simulink model "IsourceTest"  (Simulink 8.1)
settings: Solver=FixedStepDiscrete  StartTime=0.0  StopTime=2  FixedStep=Ts  RelTol=1e-3
undefined symbols (not defined in the file or in its folder): D1, Delta, DiscIntNeverNeededParam, sigbuilder_block, Ts
libraries: powerlib x8, breaker_lib x2, IsourcePower_lib x1
settings Model: Creator=pkoralew  LastModifiedBy=pkoralew
settings DebuggingCC: FcnCallInpInsideContextMsg=EnableAllAsWarning

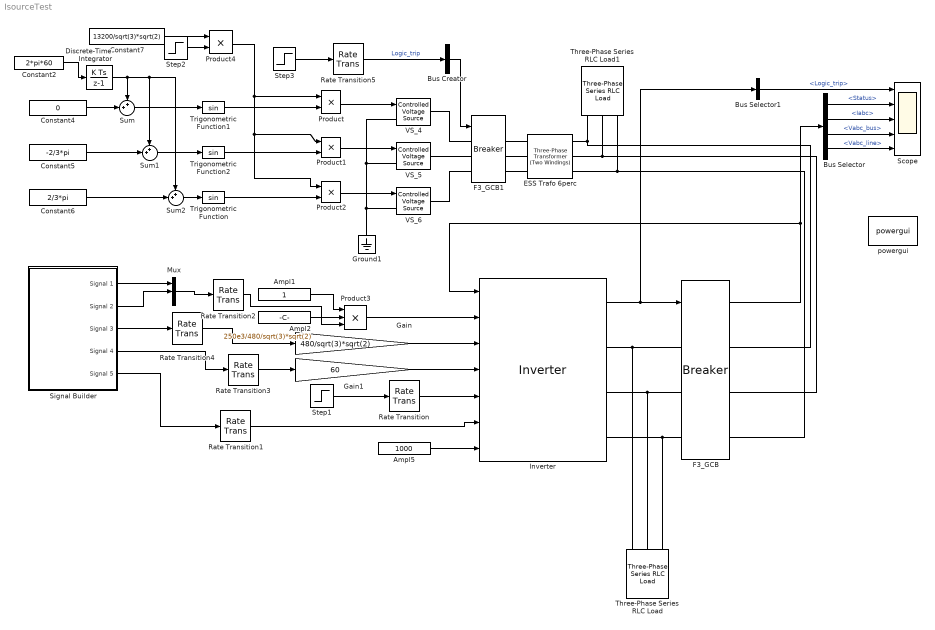
== system IsourceTest ==
  Ampl1 : Constant
  Ampl2 : Constant  Value=250e3/480/sqrt(3)*sqrt(2)
  Ampl5 : Constant  Value=1000
  Bus Creator : BusCreator  Inputs=1
  Bus Selector : BusSelector  OutputSignals=Status,Iabc,Vabc_bus,Vabc_line
  Bus Selector1 : BusSelector  OutputSignals=Logic_trip
  Constant2 : Constant  Value=2*pi*60
  Constant4 : Constant  Value=0
  Constant5 : Constant  Value=-2/3*pi
  Constant6 : Constant  Value=2/3*pi
  Constant7 : Constant  Value=13200/sqrt(3)*sqrt(2)
  Discrete-Time Integrator : DiscreteIntegrator  SampleTime=Ts  ICPrevOutput=DiscIntNeverNeededParam  ICPrevScaledInput=DiscIntNeverNeededParam
  ESS Trafo 6perc : powerlib/Elements/Three-Phase Transformer (Two Windings)  Winding1Connection=Yg  UNITS=pu  NominalPower=[250e3 60]  Winding1=[480 0.003 0.03]  Winding2Connection=Delta (D1)  Winding2=[13200 0.003 0.03]  SetSaturation=off  Rm=100  Lm=100  Saturation=[0 0;0.0031999 1.2;1.3333 1.52]  Hysteresis=off  DataFile='hysteresis'  SetInitialFlux=off  InitialFluxes=[0.79999 -0.79999 0.70002]  Measurements=Fluxes and magnetization currents ( Imag )  MoreParameters=off  BreakLoop=off  DataType=off  TransfoNumber=1
  F3_GCB : breaker_lib/Breaker  Ts=Ts  mech_delay=cb_mech_delay
  F3_GCB1 : breaker_lib/Breaker  Ts=Ts  mech_delay=cb_mech_delay
  Gain : Gain  Gain=480/sqrt(3)*sqrt(2)
  Gain1 : Gain  Gain=60
  Ground1 : powerlib/Elements/Ground  LConnTagsString=a
  Inverter : IsourcePower_lib/Inverter
  Mux : Mux  Inputs=3
  Product : Product  RndMeth=Zero
  Product1 : Product  RndMeth=Zero
  Product2 : Product  RndMeth=Zero
  Product3 : Product  Inputs=3  RndMeth=Zero
  Product4 : Product
  Rate Transition{,1..5} (6 alike) : RateTransition
  Scope : Scope  NumInputPorts=5
      settings: YMin=-5~-5~-5~-5~-5  YMax=5~5~5~5~5
  Signal Builder : Subsystem  Tag=STV Subsys  LoadFcn=sigbuilder_block('load');  StartFcn=sigbuilder_block('start');  StopFcn=sigbuilder_block('stop');  ClipboardFcn=sigbuilder_block('clipboard');  mask(Sigbuilder block){}
      mask help: Sigbuilder GUI
      mask init:
      | if ~strcmp(get_param(bdroot(gcbh),'SimulationStatus'),'stopped') tuvar = sigbuilder_block('maskInit'); end
      settings: CopyFcn=sigbuilder_block('copy');  DeleteFcn=sigbuilder_block('delete');  ModelCloseFcn=sigbuilder_block('modelClose');  PreSaveFcn=sigbuilder_block('preSave');  PauseFcn=sigbuilder_block('pause')  ContinueFcn=sigbuilder_block('continue')  NameChangeFcn=sigbuilder_block('namechange');  OpenFcn=sigbuilder_block('open',[5.58621 9.31034 1031.59 587.793 ]);  CloseFcn=sigbuilder_block('close');
      mask Display: plot(0,0,100,100,[10,10,40,40,10],[80,20,20,80,80],[40,10],[50,50], [40,27,10],[65,72,56],[40,25,25,10],[28,28,43,43]);
  Step1 : Step  SampleTime=0
  Step2 : Step  Time=0.001  SampleTime=0
  Step3 : Step  Before=1  After=0  SampleTime=0
  Sum : Sum  Inputs=++|
  Sum1 : Sum  Inputs=++|
  Sum2 : Sum  Inputs=++|
  Three-Phase Series RLC Load : powerlib/Elements/Three-Phase Series RLC Load  LConnTagsString=A|B|C  Configuration=Delta  NominalVoltage=480  NominalFrequency=60  ActivePower=1e3  InductivePower=0  CapacitivePower=100  Measurements=None  LoadType=constant Z
  Three-Phase Series RLC Load1 : powerlib/Elements/Three-Phase Series RLC Load  LConnTagsString=A|B|C  Configuration=Delta  NominalVoltage=480  NominalFrequency=60  ActivePower=1e3  InductivePower=0  CapacitivePower=100  Measurements=None  LoadType=constant Z
  Trigonometric Function : Trigonometry
  Trigonometric Function1 : Trigonometry
  Trigonometric Function2 : Trigonometry
  VS_4 : powerlib/Electrical Sources/Controlled Voltage Source  Initialize=off  Source_Type=AC  Amplitude=0  Phase=0  Frequency=0  Measurements=None
  VS_5 : powerlib/Electrical Sources/Controlled Voltage Source  Initialize=off  Source_Type=AC  Amplitude=0  Phase=0  Frequency=0  Measurements=None
  VS_6 : powerlib/Electrical Sources/Controlled Voltage Source  Initialize=off  Source_Type=AC  Amplitude=0  Phase=0  Frequency=0  Measurements=None
  powergui : powerlib/powergui  Priority=1  SimulationMode=Discrete  SolverType=Tustin  SampleTime=Ts  frequency=60  SPID=off  DisableSnubberDevices=off  DisableRonSwitches=off  DisableVfSwitches=off  SwTol=0  Interpol=off  DisplayEquations=off  frequencyindice=0  Pbase=100e6  ErrMax=1e-4  Iterations=50  UnitsV=kV  UnitsW=MW  FunctionMessages=off  echomessages=off  HookPort=off  EnableUseOfTLC=off  x0status=blocks  RestoreLinks=warning  ResistiveCurrentMeasurement=off  Frange=[0:2:500]  Ylog=off  Xlog=on  ShowGrid=off  save=off  variable=ZData  ZoomFFT=off  StartTime=0.0  cycles=1  DisplayStyle=1  fundamental=60  FreqAxis=off  MaxFrequency=1000  frequencyindicesteady=1  RmsSteady=1  display=off  Ts=0  methode=off
  wires:
  Product4/1 -> Product1/1, Product2/1, Product/1
  Trigonometric Function1/1 -> Product/2
  Discrete-Time Integrator/1 -> Sum2/1, Sum1/1, Sum/1
  Sum/1 -> Trigonometric Function1/1
  Sum1/1 -> Trigonometric Function2/1
  Constant2/1 -> Discrete-Time Integrator/1
  Constant4/1 -> Sum/2
  Sum2/1 -> Trigonometric Function/1
  Constant5/1 -> Sum1/2
  Constant6/1 -> Sum2/2
  Trigonometric Function2/1 -> Product1/2
  Trigonometric Function/1 -> Product2/2
  Product/1 -> VS_4/1
  Product1/1 -> VS_5/1
  Product2/1 -> VS_6/1
  Ampl2/1 -> Product3/2
  Ampl1/1 -> Product3/1
  Product3/1 -> Inverter/2
  Signal Builder/5(Signal 5) -> Rate Transition1/1
  Step1/1 -> Rate Transition/1
  Gain1/1 -> Inverter/4
  Constant7/1 -> Product4/1
  Step2/1 -> Product4/2
  Inverter/1 -> Bus Selector1/1, F3_GCB/1
  F3_GCB/1 -> Bus Selector/1, Inverter/1
  Bus Selector1/1 -> Scope/1  "<Logic_trip>"
  Bus Selector/2 -> Scope/3  "<Iabc>"
  Bus Selector/1 -> Scope/2  "<Status>"
  Bus Selector/4 -> Scope/5  "<Vabc_line>"
  Bus Selector/3 -> Scope/4  "<Vabc_bus>"
  Rate Transition/1 -> Inverter/5
  Rate Transition1/1 -> Inverter/6
  Rate Transition2/1 -> Product3/3
  Ampl5/1 -> Inverter/7
  Gain/1 -> Inverter/3
  Mux/1 -> Rate Transition2/1
  Signal Builder/1(Signal 1) -> Mux/1
  Signal Builder/2(Signal 2) -> Mux/2
  Signal Builder/3(Signal 3) -> Rate Transition4/1
  Signal Builder/4(Signal 4) -> Rate Transition3/1
  Rate Transition3/1 -> Gain1/1
  Rate Transition4/1 -> Gain/1
  Rate Transition5/1 -> Bus Creator/1  "Logic_trip"
  Step3/1 -> Rate Transition5/1
  Bus Creator/1 -> F3_GCB1/1
  connections:
  Ground1/LConn1 -- VS_6/LConn1 -- VS_5/LConn1 -- VS_4/LConn1
  ESS Trafo 6perc/LConn2 -- F3_GCB/RConn2 -- Three-Phase Series RLC Load1/LConn2
  ESS Trafo 6perc/LConn3 -- F3_GCB/RConn3 -- Three-Phase Series RLC Load1/LConn3
  ESS Trafo 6perc/LConn1 -- F3_GCB/RConn1 -- Three-Phase Series RLC Load1/LConn1
  Three-Phase Series RLC Load/LConn1 -- Inverter/RConn1 -- F3_GCB/LConn1
  Three-Phase Series RLC Load/LConn2 -- Inverter/RConn2 -- F3_GCB/LConn2
  Three-Phase Series RLC Load/LConn3 -- Inverter/RConn3 -- F3_GCB/LConn3
  VS_4/RConn1 -- F3_GCB1/LConn1
  F3_GCB1/LConn2 -- VS_5/RConn1
  F3_GCB1/LConn3 -- VS_6/RConn1
  F3_GCB1/RConn1 -- ESS Trafo 6perc/RConn1
  F3_GCB1/RConn2 -- ESS Trafo 6perc/RConn2
  F3_GCB1/RConn3 -- ESS Trafo 6perc/RConn3

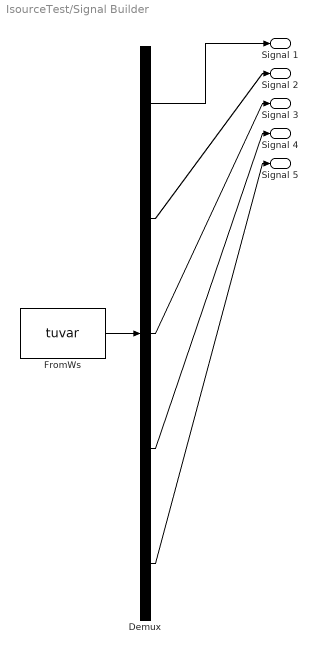
== system IsourceTest/Signal Builder ==
  Demux : Demux  Tag=STV Demux  Outputs=5
  FromWs : FromWorkspace  Tag=STV FromWs  VariableName=tuvar  SampleTime=0  SigBuilderData=DataTag0  VnvData=DataTag1
      SigBuilderData=|
      | common.afterFinalStr = 'Extrapolate'
      | common.sampleTime = 0
      | dataSet(1).timeRange = [0 2]
      | dataSet(1).name = 'Group 2'
      | dataSet(2).timeRange = [0 0.4]
      | dataSet(2).name = 'Group 3'
      | dataSet(3).timeRange = [0 0.4]
      | dataSet(3).name = 'Group 4'
      | dataSet(4).timeRange = [0 0.4]
      | dataSet(4).name = 'Group 5'
      | dataSet(5).timeRange = [0 0.4]
      | dataSet(5).name = 'Group 6'
      | sbobj.Groups(1).Name = 'Group 2'
      | sbobj.Groups(1).Signals(1).Name = 'Signal 1'
      | sbobj.Groups(1).Signals(1).XData = [0 0.3 0.385 0.455 0.532 0.634 0.634 0.746 0.746 0.85 2]
      | sbobj.Groups(1).Signals(1).YData = [0 0 1 1 0 0 -1 -1 0 0 0]
      | sbobj.Groups(1).Signals(2).Name = 'Signal 2'
      | sbobj.Groups(1).Signals(2).XData = [0 0.33 0.5 0.59 0.7 0.806 2]
      | sbobj.Groups(1).Signals(2).YData = [0 0 1 1 -1 0 0]
      | sbobj.Groups(1).Signals(3).Name = 'Signal 3'
      | sbobj.Groups(1).Signals(3).XData = [0 1 1 1.202 1.202 2]
      | sbobj.Groups(1).Signals(3).YData = [1 1 0.71 0.71 1.39 1.39]
      | sbobj.Groups(1).Signals(4).Name = 'Signal 4'
      | sbobj.Groups(1).Signals(4).XData = [0 1.202 1.202 1.396 1.396 2]
      | sbobj.Groups(1).Signals(4).YData = [1 1 0.95 0.95 1.048 1.048]
      | sbobj.Groups(1).Signals(5).Name = 'Signal 5'
      | sbobj.Groups(1).Signals(5).XData = [0 0.042 0.042 1.488 1.488 1.636 1.636 2]
      | sbobj.Groups(1).Signals(5).YData = [0 0 1 1 0 0 1 1]
      | sbobj.Groups(1).TimeRange = [0 2]
      | sbobj.Groups(2).Name = 'Group 3'
      | sbobj.Groups(2).Signals(1).Name = 'Signal 1'
      | sbobj.Groups(2).Signals(1).XData = [0 0.005 0.03 0.041 0.0445 0.0575 0.0675 0.0785 0.0905 0.0945 0.1055 0.1115 0.133 0.1455 0.1565 0.1635 0.192 0.218 0.306 0.3075 0.4]
      | sbobj.Groups(2).Signals(1).YData = [0 0 0.5 0.5 0.382 0.384 0.7 0.702 0.918 0.482 0.482 1 1 0.606 0.74 0.35 0.672 0.014 0.398 0.202 0]
      | sbobj.Groups(2).Signals(2).Name = 'Signal 2'
      | sbobj.Groups(2).Signals(2).XData = [0 0.16 0.16 0.24 0.24 10]
      | sbobj.Groups(2).Signals(2).YData = [0 0 1 1 0 0]
      | sbobj.Groups(2).Signals(3).Name = 'Signal 3'
      | sbobj.Groups(2).Signals(3).XData = [0 1 1 10]
      | sbobj.Groups(2).Signals(3).YData = [0 0 1 1]
      | sbobj.Groups(2).Signals(4).Name = 'Signal 4'
      | sbobj.Groups(2).Signals(4).XData = [0 1 1 10]
      | sbobj.Groups(2).Signals(4).YData = [0 0 1 1]
      | sbobj.Groups(2).Signals(5).Name = 'Signal 5'
      | sbobj.Groups(2).Signals(5).XData = [0 1 1 10]
      | sbobj.Groups(2).Signals(5).YData = [0 0 1 1]
      | sbobj.Groups(3).Name = 'Group 4'
      | sbobj.Groups(3).Signals(1).Name = 'Signal 1'
      | sbobj.Groups(3).Signals(1).XData = [0 0.1 0.1 0.2 0.2 0.4]
      | sbobj.Groups(3).Signals(1).YData = [0 0 0.5 0.5 0 0]
      | sbobj.Groups(3).Signals(2).Name = 'Signal 2'
      | sbobj.Groups(3).Signals(2).XData = [0 0.16 0.16 0.24 0.24 10]
      | sbobj.Groups(3).Signals(2).YData = [0 0 1 1 0 0]
      | sbobj.Groups(3).Signals(3).Name = 'Signal 3'
      | sbobj.Groups(3).Signals(3).XData = [0 1 1 10]
      | sbobj.Groups(3).Signals(3).YData = [0 0 1 1]
      | sbobj.Groups(3).Signals(4).Name = 'Signal 4'
      | sbobj.Groups(3).Signals(4).XData = [0 1 1 10]
      | sbobj.Groups(3).Signals(4).YData = [0 0 1 1]
      | sbobj.Groups(3).Signals(5).Name = 'Signal 5'
      | sbobj.Groups(3).Signals(5).XData = [0 1 1 10]
      | sbobj.Groups(3).Signals(5).YData = [0 0 1 1]
      | sbobj.Groups(4).Name = 'Group 5'
      | sbobj.Groups(4).Signals(1).Name = 'Signal 1'
      | sbobj.Groups(4).Signals(1).XData = [0 0.02 0.05 0.4]
      | sbobj.Groups(4).Signals(1).YData = [0 -0.001 0.5 0.5]
      | sbobj.Groups(4).Signals(2).Name = 'Signal 2'
      | sbobj.Groups(4).Signals(2).XData = [0 0.16 0.16 0.24 0.24 10]
      | sbobj.Groups(4).Signals(2).YData = [0 0 1 1 0 0]
      | sbobj.Groups(4).Signals(3).Name = 'Signal 3'
      | sbobj.Groups(4).Signals(3).XData = [0 1 1 10]
      | sbobj.Groups(4).Signals(3).YData = [0 0 1 1]
      | sbobj.Groups(4).Signals(4).Name = 'Signal 4'
      | sbobj.Groups(4).Signals(4).XData = [0 1 1 10]
      | sbobj.Groups(4).Signals(4).YData = [0 0 1 1]
      | sbobj.Groups(4).Signals(5).Name = 'Signal 5'
      | sbobj.Groups(4).Signals(5).XData = [0 1 1 10]
      | sbobj.Groups(4).Signals(5).YData = [0 0 1 1]
      | sbobj.Groups(5).Name = 'Group 6'
      | sbobj.Groups(5).Signals(1).Name = 'Signal 1'
      | sbobj.Groups(5).Signals(1).XData = [0 0.4]
      | sbobj.Groups(5).Signals(1).YData = [0.05 0.05]
      | sbobj.Groups(5).Signals(2).Name = 'Signal 2'
      | sbobj.Groups(5).Signals(2).XData = [0 0.16 0.16 0.24 0.24 10]
      | sbobj.Groups(5).Signals(2).YData = [0 0 1 1 0 0]
      | sbobj.Groups(5).Signals(3).Name = 'Signal 3'
      | sbobj.Groups(5).Signals(3).XData = [0 1 1 10]
      | sbobj.Groups(5).Signals(3).YData = [0 0 1 1]
      | sbobj.Groups(5).Signals(4).Name = 'Signal 4'
      | sbobj.Groups(5).Signals(4).XData = [0 1 1 10]
      | sbobj.Groups(5).Signals(4).YData = [0 0 1 1]
      | sbobj.Groups(5).Signals(5).Name = 'Signal 5'
      | sbobj.Groups(5).Signals(5).XData = [0 1 1 10]
      | sbobj.Groups(5).Signals(5).YData = [0 0 1 1]
  Signal 1 : Outport  Tag=STV Outport
  Signal 2 : Outport  Tag=STV Outport  Port=2
  Signal 3 : Outport  Tag=STV Outport  Port=3
  Signal 4 : Outport  Tag=STV Outport  Port=4
  Signal 5 : Outport  Tag=STV Outport  Port=5
  wires:
  Demux/1 -> Signal 1/1
  FromWs/1 -> Demux/1
  Demux/2 -> Signal 2/1
  Demux/3 -> Signal 3/1
  Demux/4 -> Signal 4/1
  Demux/5 -> Signal 5/1
